simulink model "smm_gait_control"  (R2018b)
settings: configuration reference "Configuration1khz" (kept outside this file)
InitFcn:
  | addpath('./functions/')
  | addpath('./policies/')
  | control_params
values from neighbouring files (symbols this model uses):
  rest = extract_policy_variables('policies/rest.mat')    [control_params.m]
  run_slow = extract_policy_variables('policies/06_run_reduced.mat')    [control_params.m]
  walk_slow = extract_policy_variables('policies/06_walk.mat')    [control_params.m]
undefined symbols (not defined in the file or in its folder): ctrl, Discrete, initial_dx_estimate, initial_dy_estimate, initial_dz_estimate, initial_z_estimate, sample_time, Time
libraries: simulink x42, ctrlSharedLib x7
(part 3 of 5)

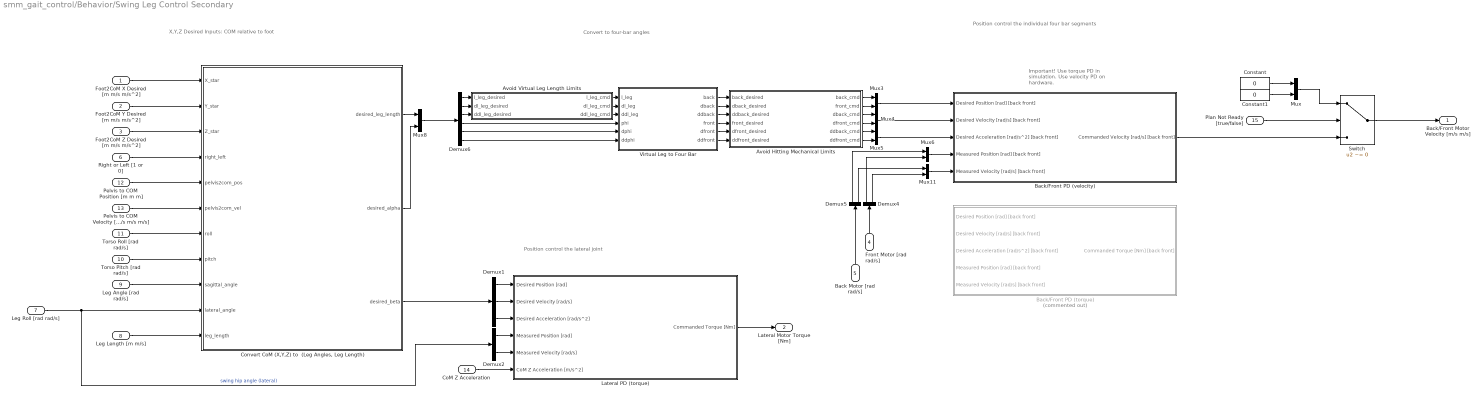
== system smm_gait_control/Behavior/Swing Leg Control Secondary ==
  note: Position control the
      | individual four bar segments
  note: Convert to four-bar angles
  note: X,Y,Z Desired Inputs: COM relative to foot
  note: Important!
      | Use torque PD in simulation.
      | Use velocity PD on hardware.
  note: Position control the lateral joint
  Foot2CoM X Desired [m m/s m/s^2] : Inport
  Foot2CoM Y Desired [m m/s m/s^2] : Inport  Port=2
  Foot2CoM Z Desired [m m/s m/s^2] : Inport  Port=3
  Front Motor [rad rad/s] : Inport  Port=4
  Back Motor [rad rad/s] : Inport  Port=5
  Right or Left [1 or 0] : Inport  Port=6
  Leg Roll [rad rad/s] : Inport  Port=7
  Leg Length [m m/s] : Inport  Port=8
  Leg Angle [rad rad/s] : Inport  Port=9
  Torso Pitch [rad rad/s] : Inport  Port=10
  Torso Roll [rad rad/s] : Inport  Port=11
  Pelvis to COM Position [m m m] : Inport  Port=12
  Pelvis to COM Velocity [m/s m/s m/s] : Inport  Port=13
  CoM Z Acceleration : Inport  Port=14
  Plan Not Ready [true/false] : Inport  Port=15
  Avoid Hitting Mechanical Limits : MATLAB Function  TreatAsAtomicUnit=on
  Avoid Virtual Leg Length Limits : MATLAB Function  TreatAsAtomicUnit=on
  Back/Front PD (torque) : Subsystem  Commented=on
  Back/Front PD (velocity) : Subsystem
  Constant : Constant  Value=0
  Constant1 : Constant  Value=0
  "Convert CoM (X,Y,Z) to  (Leg Angles, Leg Length)" : MATLAB Function  TreatAsAtomicUnit=on
  Demux1 : Demux  Outputs=3
  Demux2 : Demux  Outputs=2
  Demux4 : Demux  Outputs=2
  Demux5 : Demux  Outputs=2
  Demux6 : Demux  Outputs=6
  Lateral PD (torque) : Subsystem
  Mux{,3..6,8,11} (7 alike) : Mux  Inputs=2
  Switch : Switch  Criteria=u2 ~= 0
  Virtual Leg to Four Bar : MATLAB Function  TreatAsAtomicUnit=on
  Back/Front Motor Velocity [m/s m/s] : Outport
  Lateral Motor Torque [Nm] : Outport  Port=2
  wires:
  Demux4/1 -> Mux6/2
  Mux6/1 -> Back/Front PD (velocity)/4(Measured Position [rad] [back front])
  Mux3/1 -> Back/Front PD (velocity)/1(Desired Position [rad] [back front])
  Demux5/2 -> Mux11/1
  Front Motor [rad rad/s]/1 -> Demux4/1
  Mux4/1 -> Back/Front PD (velocity)/2(Desired Velocity [rad/s] [back front])
  Foot2CoM Z Desired [m m/s m/s^2]/1 -> "Convert CoM (X,Y,Z) to  (Leg Angles, Leg Length)"/3(Z_star)
  Demux5/1 -> Mux6/1
  Back Motor [rad rad/s]/1 -> Demux5/1
  Demux6/4 -> Virtual Leg to Four Bar/4(phi)
  Mux11/1 -> Back/Front PD (velocity)/5(Measured Velocity [rad/s] [back front])
  Demux6/6 -> Virtual Leg to Four Bar/6(ddphi)
  Demux6/5 -> Virtual Leg to Four Bar/5(dphi)
  Demux4/2 -> Mux11/2
  Torso Pitch [rad rad/s]/1 -> "Convert CoM (X,Y,Z) to  (Leg Angles, Leg Length)"/8(pitch)
  Torso Roll [rad rad/s]/1 -> "Convert CoM (X,Y,Z) to  (Leg Angles, Leg Length)"/7(roll)
  Right or Left [1 or 0]/1 -> "Convert CoM (X,Y,Z) to  (Leg Angles, Leg Length)"/4(right_left)
  Leg Roll [rad rad/s]/1 -> Demux2/1, "Convert CoM (X,Y,Z) to  (Leg Angles, Leg Length)"/10(lateral_angle)  "swing hip angle (lateral)"
  Leg Angle [rad rad/s]/1 -> "Convert CoM (X,Y,Z) to  (Leg Angles, Leg Length)"/9(sagittal_angle)
  "Convert CoM (X,Y,Z) to  (Leg Angles, Leg Length)"/2(desired_alpha) -> Mux8/2
  Leg Length [m m/s]/1 -> "Convert CoM (X,Y,Z) to  (Leg Angles, Leg Length)"/11(leg_length)
  "Convert CoM (X,Y,Z) to  (Leg Angles, Leg Length)"/1(desired_leg_length) -> Mux8/1
  Mux8/1 -> Demux6/1
  Foot2CoM Y Desired [m m/s m/s^2]/1 -> "Convert CoM (X,Y,Z) to  (Leg Angles, Leg Length)"/2(Y_star)
  Pelvis to COM Position [m m m]/1 -> "Convert CoM (X,Y,Z) to  (Leg Angles, Leg Length)"/5(pelvis2com_pos)
  Pelvis to COM Velocity [m/s m/s m/s]/1 -> "Convert CoM (X,Y,Z) to  (Leg Angles, Leg Length)"/6(pelvis2com_vel)
  "Convert CoM (X,Y,Z) to  (Leg Angles, Leg Length)"/3(desired_beta) -> Demux1/1
  Foot2CoM X Desired [m m/s m/s^2]/1 -> "Convert CoM (X,Y,Z) to  (Leg Angles, Leg Length)"/1(X_star)
  Mux5/1 -> Back/Front PD (velocity)/3(Desired Acceleration [rad/s^2] [back front])
  Demux1/1 -> Lateral PD (torque)/1(Desired Position [rad])
  Demux1/3 -> Lateral PD (torque)/3(Desired Acceleration [rad/s^2])
  Demux1/2 -> Lateral PD (torque)/2(Desired Velocity [rad/s])
  Lateral PD (torque)/1(Commanded Torque [Nm]) -> Lateral Motor Torque [Nm]/1
  Demux2/2 -> Lateral PD (torque)/5(Measured Velocity [rad/s])
  Demux2/1 -> Lateral PD (torque)/4(Measured Position [rad])
  CoM Z Acceleration/1 -> Lateral PD (torque)/6(CoM Z Acceleration [m/s^2])
  Virtual Leg to Four Bar/1(back) -> Avoid Hitting Mechanical Limits/1(back_desired)
  Virtual Leg to Four Bar/2(dback) -> Avoid Hitting Mechanical Limits/2(dback_desired)
  Virtual Leg to Four Bar/3(ddback) -> Avoid Hitting Mechanical Limits/3(ddback_desired)
  Virtual Leg to Four Bar/4(front) -> Avoid Hitting Mechanical Limits/4(front_desired)
  Virtual Leg to Four Bar/5(dfront) -> Avoid Hitting Mechanical Limits/5(dfront_desired)
  Virtual Leg to Four Bar/6(ddfront) -> Avoid Hitting Mechanical Limits/6(ddfront_desired)
  Avoid Hitting Mechanical Limits/1(back_cmd) -> Mux3/1
  Avoid Hitting Mechanical Limits/6(ddfront_cmd) -> Mux5/2
  Avoid Hitting Mechanical Limits/2(front_cmd) -> Mux3/2
  Avoid Hitting Mechanical Limits/3(dback_cmd) -> Mux4/1
  Avoid Hitting Mechanical Limits/4(dfront_cmd) -> Mux4/2
  Avoid Hitting Mechanical Limits/5(ddback_cmd) -> Mux5/1
  Demux6/1 -> Avoid Virtual Leg Length Limits/1(l_leg_desired)
  Demux6/2 -> Avoid Virtual Leg Length Limits/2(dl_leg_desired)
  Demux6/3 -> Avoid Virtual Leg Length Limits/3(ddl_leg_desired)
  Avoid Virtual Leg Length Limits/1(l_leg_cmd) -> Virtual Leg to Four Bar/1(l_leg)
  Avoid Virtual Leg Length Limits/2(dl_leg_cmd) -> Virtual Leg to Four Bar/2(dl_leg)
  Avoid Virtual Leg Length Limits/3(ddl_leg_cmd) -> Virtual Leg to Four Bar/3(ddl_leg)
  Mux/1 -> Switch/1
  Constant/1 -> Mux/1
  Back/Front PD (velocity)/1(Commanded Velocity [rad/s] [back front]) -> Switch/3
  Plan Not Ready [true/false]/1 -> Switch/2
  Constant1/1 -> Mux/2
  Switch/1 -> Back/Front Motor Velocity [m/s m/s]/1

== system smm_gait_control/Behavior/Tranform Sensor Measurements to CoM Acceleration Measurement ==
  note: Important!
      | Include gravitational acceleration.
      | (Not measured by accelerometers)
  Pitch State [rad rad/s] : Inport
  Roll State [rad rad/s] : Inport  Port=2
  Yaw State [rad rad/s] : Inport  Port=3
  Imu Accelerations : Inport  Port=4
  Enabled [true/false] : Inport  Port=5
  R Hip Roll [rad rad/s] : Inport  Port=6
  L Hip Roll [rad rad/s] : Inport  Port=7
  COM Acceleration Measurement : Scope  NumInputPorts=3
  Compute Body Frame Accelerations : Subsystem
  Compute CoM Translational Acceleration : MATLAB Function  TreatAsAtomicUnit=on
  Demux : Demux  Outputs=3
  Demux3 : Demux  Outputs=3
  Estimate Angular Accelerations2 : Subsystem
  Estimate Angular Accelerations3 : Subsystem
  Fcn : Fcn  Expr=u - ctrl.g
  Mux28 : Mux  Inputs=3
  Mux3 : Mux  Inputs=3
  Mux30 : Mux  Inputs=2
  Selector{,1..2,41..42} (5 alike) : Selector  InputPortWidth=2  IndexOptions=Index vector (dialog)  Indices=[2]  OutputSizes=1
  Terminator{3..5,7} (4 alike) : Terminator
  CoM Acceleration [m/s] x3 : Outport
  wires:
  Demux/1 -> COM Acceleration Measurement/1
  Demux/3 -> COM Acceleration Measurement/3
  [enabled] -> Estimate Angular Accelerations2/2(Enabled)
  Yaw State [rad rad/s]/1 -> Selector2/1
  Mux30/1 -> Estimate Angular Accelerations3/1(Angular Velocities [rad/s] x2)
  Demux/2 -> COM Acceleration Measurement/2
  Pitch State [rad rad/s]/1 -> Selector1/1, Compute CoM Translational Acceleration/4(torso_pitch)
  Roll State [rad rad/s]/1 -> Selector/1, Compute CoM Translational Acceleration/3(torso_roll)
  Estimate Angular Accelerations2/1(Angular Accelerations [rad/s^2] x3) -> Compute CoM Translational Acceleration/1(torso_angular_accelerations)
  Compute Body Frame Accelerations/1(accelerations [m/s^2] x3) -> Compute CoM Translational Acceleration/2(imu_translational_accelerations_body)
  Compute CoM Translational Acceleration/5(left_hip_acceleration_yawed) -> Terminator5/1
  Compute CoM Translational Acceleration/2(torso_com_acceleration_yawed) -> Terminator3/1
  Mux28/1 -> Estimate Angular Accelerations2/1(Angular Velocities [rad/s] x3)
  Imu Accelerations/1 -> Compute Body Frame Accelerations/1(imu accelerations x3)
  R Hip Roll [rad rad/s]/1 -> Selector41/1, Compute CoM Translational Acceleration/6(right_hip_roll)
  L Hip Roll [rad rad/s]/1 -> Selector42/1, Compute CoM Translational Acceleration/7(left_hip_roll)
  Selector/1 -> Mux28/1
  Selector1/1 -> Mux28/2
  Selector2/1 -> Mux28/3
  Compute CoM Translational Acceleration/4(right_hip_acceleration_yawed) -> Terminator4/1
  Compute CoM Translational Acceleration/3(pelvis_acceleration_yawed) -> Terminator7/1
  Demux3/1 -> Mux3/1
  Demux3/3 -> Fcn/1
  Fcn/1 -> Mux3/3
  Demux3/2 -> Mux3/2
  Compute CoM Translational Acceleration/1(com_acceleration_yawed) -> Demux3/1
  Selector41/1 -> Mux30/1
  Selector42/1 -> Mux30/2
  Estimate Angular Accelerations3/1(Angular Accelerations [rad/s^2] x2) -> Compute CoM Translational Acceleration/5(hip_roll_accelerations)
  Enabled [true/false]/1 -> [enabled]
  [enabled] -> Estimate Angular Accelerations3/2(Enabled)
  Mux3/1 -> Demux/1, CoM Acceleration [m/s] x3/1

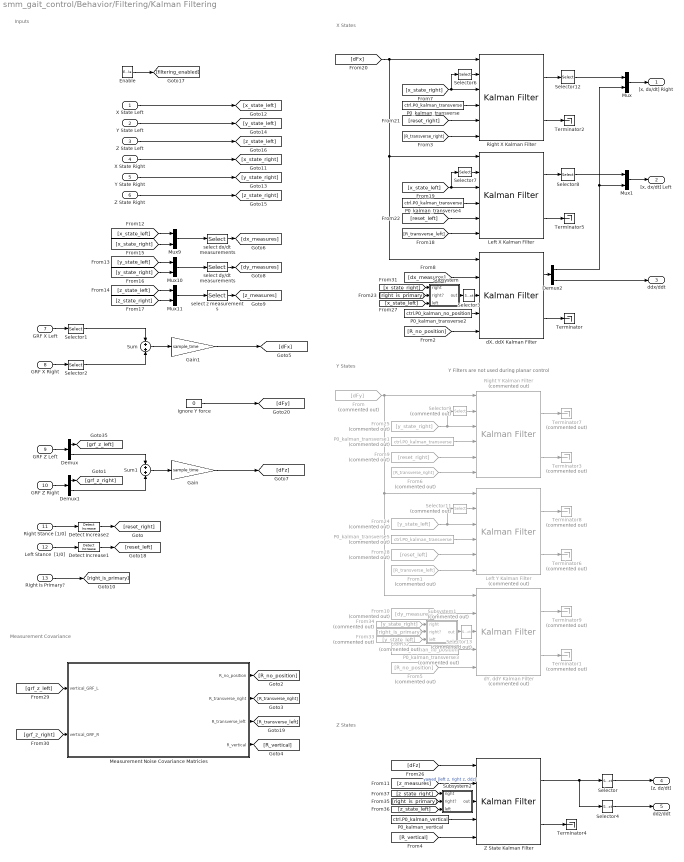
== system smm_gait_control/Behavior/Filtering/Kalman Filtering ==
  note: Y Filters are not used during planar control
  note: Inputs
  note: X States
  note: Y States
  note: Z States
  note: Measurement Covariance
  X State Left : Inport  SampleTime=sample_time
  Y State Left : Inport  Port=2  SampleTime=sample_time
  Z State Left : Inport  Port=3  SampleTime=sample_time
  X State Right : Inport  Port=4  SampleTime=sample_time
  Y State Right : Inport  Port=5  SampleTime=sample_time
  Z State Right : Inport  Port=6  SampleTime=sample_time
  GRF X Left : Inport  Port=7  SampleTime=sample_time
  GRF X Right : Inport  Port=8  SampleTime=sample_time
  GRF Z Left : Inport  Port=9  SampleTime=sample_time
  GRF Z Right : Inport  Port=10  SampleTime=sample_time
  Right Stance [1/0] : Inport  Port=11  PortDimensions=1  SampleTime=sample_time
  Left Stance  [1/0] : Inport  Port=12  PortDimensions=1  SampleTime=sample_time
  Right Is Primary? : Inport  Port=13  SampleTime=sample_time
  Enable : EnablePort  StatesWhenEnabling=reset  ShowOutputPort=on
  Demux : Demux  Outputs=2
  Demux1 : Demux  Outputs=2
  Demux2 : Demux  Outputs=2
  Detect Increase1 : simulink/Logic and Bit Operations/Detect Increase  vinit=0.0  OutDataTypeStr=boolean
  Detect Increase2 : simulink/Logic and Bit Operations/Detect Increase  vinit=0.0  OutDataTypeStr=boolean
  From : From  Commented=on  GotoTag=dFy
  From1 : From  Commented=on  GotoTag=R_transverse_left
  From10 : From  Commented=on  GotoTag=dy_measures
  From24 : From  Commented=on  GotoTag=y_state_left
  From25 : From  Commented=on  GotoTag=y_state_right
  From28 : From  Commented=on  GotoTag=reset_left
  From32 : From  Commented=on  GotoTag=right_is_primary
  From33 : From  Commented=on  GotoTag=y_state_left
  From34 : From  Commented=on  GotoTag=y_state_right
  From5 : From  Commented=on  GotoTag=R_no_position
  From6 : From  Commented=on  GotoTag=R_transverse_right
  From9 : From  Commented=on  GotoTag=reset_right
  Gain : Gain  Gain=sample_time
  Gain1 : Gain  Gain=sample_time
  Ignore Y force : Constant  Value=0
  Left X Kalman Filter : ctrlSharedLib/Kalman Filter  TimeDomain=Discrete-Time  UseCurrentEstimator=on  ModelSource=Individual A, B, C, D matrices  ModelSourceVariable=A_kf  A=ctrl.A_kalman_3rd_order  B=ctrl.B_kalman_3rd_order  C=ctrl.C_kalman_transverse  D=0  NumberOfStates=2  NumberOfInputs=1  NumberOfOutputs=2  InitialEstimateSource=Input port  X0=initial_dx_estimate  P0=P0_kalman_transverse  UseK=off  UseGH=on  NumberOfProcessNoiseInputs=1  G=ctrl.G_kalman_transverse  TimeInvariantG=on  H=0  TimeInvariantH=on  Q=ctrl.Q_kalman_GRFx_difference*sample_time  TimeInvariantQ=on  R=1  TimeInvariantR=off  N=0  TimeInvariantN=on  AddInputPort=on  AddEnablePort=off  ExternalReset=Rising  OutputEstimatedY=off  OutputP=on  Ts=sample_time
      settings: SourceProductBaseCode=CT
  Left Y Kalman Filter : ctrlSharedLib/Kalman Filter  Commented=on  TimeDomain=Discrete-Time  UseCurrentEstimator=on  ModelSource=Individual A, B, C, D matrices  ModelSourceVariable=A_kf  A=ctrl.A_kalman_3rd_order  B=ctrl.B_kalman_3rd_order  C=ctrl.C_kalman_transverse  D=0  NumberOfStates=2  NumberOfInputs=1  NumberOfOutputs=2  InitialEstimateSource=Input port  X0=initial_dy_estimate  P0=P0_kalman_transverse  UseK=off  UseGH=on  NumberOfProcessNoiseInputs=1  G=ctrl.G_kalman_transverse  TimeInvariantG=on  H=0  TimeInvariantH=on  Q=ctrl.Q_kalman_GRFy_difference*sample_time  TimeInvariantQ=on  R=1  TimeInvariantR=off  N=0  TimeInvariantN=on  AddInputPort=on  AddEnablePort=off  ExternalReset=Rising  OutputEstimatedY=off  OutputP=on  Ts=sample_time
      settings: SourceProductBaseCode=CT
  Measurement Noise Covariance Matricies : MATLAB Function  TreatAsAtomicUnit=on
  Mux{,1,9..11} (5 alike) : Mux  Inputs=2
  P0_kalman_transverse : Constant  Value=ctrl.P0_kalman_transverse
  P0_kalman_transverse1 : Constant  Commented=on  Value=ctrl.P0_kalman_transverse
  P0_kalman_transverse2 : Constant  Value=ctrl.P0_kalman_no_position
  P0_kalman_transverse3 : Constant  Commented=on  Value=ctrl.P0_kalman_no_position
  P0_kalman_transverse4 : Constant  Value=ctrl.P0_kalman_transverse
  P0_kalman_transverse5 : Constant  Commented=on  Value=ctrl.P0_kalman_transverse
  P0_kalman_vertical : Constant  Value=ctrl.P0_kalman_vertical
  Right X Kalman Filter : ctrlSharedLib/Kalman Filter  TimeDomain=Discrete-Time  UseCurrentEstimator=on  ModelSource=Individual A, B, C, D matrices  ModelSourceVariable=A_kf  A=ctrl.A_kalman_3rd_order  B=ctrl.B_kalman_3rd_order  C=ctrl.C_kalman_transverse  D=0  NumberOfStates=2  NumberOfInputs=1  NumberOfOutputs=2  InitialEstimateSource=Input port  X0=initial_dx_estimate  P0=P0_kalman_transverse  UseK=off  UseGH=on  NumberOfProcessNoiseInputs=1  G=ctrl.G_kalman_transverse  TimeInvariantG=on  H=0  TimeInvariantH=on  Q=ctrl.Q_kalman_GRFx_difference*sample_time  TimeInvariantQ=on  R=1  TimeInvariantR=off  N=0  TimeInvariantN=on  AddInputPort=on  AddEnablePort=off  ExternalReset=Rising  OutputEstimatedY=off  OutputP=on  Ts=sample_time
      settings: SourceProductBaseCode=CT
  Right Y Kalman Filter : ctrlSharedLib/Kalman Filter  Commented=on  TimeDomain=Discrete-Time  UseCurrentEstimator=on  ModelSource=Individual A, B, C, D matrices  ModelSourceVariable=A_kf  A=ctrl.A_kalman_3rd_order  B=ctrl.B_kalman_3rd_order  C=ctrl.C_kalman_transverse  D=0  NumberOfStates=2  NumberOfInputs=1  NumberOfOutputs=2  InitialEstimateSource=Input port  X0=initial_dy_estimate  P0=P0_kalman_transverse  UseK=off  UseGH=on  NumberOfProcessNoiseInputs=1  G=ctrl.G_kalman_transverse  TimeInvariantG=on  H=0  TimeInvariantH=on  Q=ctrl.Q_kalman_GRFy_difference*sample_time  TimeInvariantQ=on  R=1  TimeInvariantR=off  N=0  TimeInvariantN=on  AddInputPort=on  AddEnablePort=off  ExternalReset=Rising  OutputEstimatedY=off  OutputP=on  Ts=sample_time
      settings: SourceProductBaseCode=CT
  Selector : Selector  InputPortWidth=3  IndexOptions=Index vector (dialog)  Indices=[1 2]  OutputSizes=1
  Selector1 : Selector  InputPortWidth=2  IndexOptions=Index vector (dialog)  Indices=[2]  OutputSizes=1
  Selector11 : Selector  Commented=on  InputPortWidth=3  IndexOptions=Index vector (dialog)  Indices=[1 3]  OutputSizes=1
  Selector12 : Selector  InputPortWidth=3  IndexOptions=Index vector (dialog)  Indices=[1]  OutputSizes=1
  Selector13 : Selector  Commented=on  InputPortWidth=3  IndexOptions=Index vector (dialog)  Indices=[2 3]  OutputSizes=1
  Selector2 : Selector  InputPortWidth=2  IndexOptions=Index vector (dialog)  Indices=[2]  OutputSizes=1
  Selector3 : Selector  InputPortWidth=3  IndexOptions=Index vector (dialog)  Indices=[2 3]  OutputSizes=1
  Selector4 : Selector  InputPortWidth=3  IndexOptions=Index vector (dialog)  Indices=[3]  OutputSizes=1
  Selector6 : Selector  InputPortWidth=3  IndexOptions=Index vector (dialog)  Indices=[1 3]  OutputSizes=1
  Selector7 : Selector  InputPortWidth=3  IndexOptions=Index vector (dialog)  Indices=[1 3]  OutputSizes=1
  Selector8 : Selector  InputPortWidth=3  IndexOptions=Index vector (dialog)  Indices=[1]  OutputSizes=1
  Selector9 : Selector  Commented=on  InputPortWidth=3  IndexOptions=Index vector (dialog)  Indices=[1 3]  OutputSizes=1
  Subsystem : Subsystem
  Subsystem1 : Subsystem  Commented=on
  Subsystem2 : Subsystem
  Sum : Sum  Inputs=+|+
  Sum1 : Sum  Inputs=+|+
  Terminator{,2,4..5} (4 alike) : Terminator
  Terminator{1,3,6..9} (6 alike) : Terminator  Commented=on
  Z State Kalman Filter : ctrlSharedLib/Kalman Filter  TimeDomain=Discrete-Time  UseCurrentEstimator=on  ModelSource=Individual A, B, C, D matrices  ModelSourceVariable=A_kf  A=ctrl.A_kalman_3rd_order  B=ctrl.B_kalman_3rd_order  C=ctrl.C_kalman_vertical  D=0  NumberOfStates=2  NumberOfInputs=1  NumberOfOutputs=2  InitialEstimateSource=Input port  X0=[initial_z_estimate; initial_dz_estimate]  P0=P0_kalman_vertical  UseK=off  UseGH=on  NumberOfProcessNoiseInputs=1  G=ctrl.G_kalman_vertical  TimeInvariantG=on  H=0  TimeInvariantH=on  Q=ctrl.Q_kalman_GRFz_difference*sample_time  TimeInvariantQ=on  R=1  TimeInvariantR=off  N=0  TimeInvariantN=on  AddInputPort=on  AddEnablePort=off  OutputEstimatedY=off  OutputP=on  Ts=sample_time
      settings: SourceProductBaseCode=CT
  "dX, ddX Kalman Filter" : ctrlSharedLib/Kalman Filter  TimeDomain=Discrete-Time  UseCurrentEstimator=on  ModelSource=Individual A, B, C, D matrices  ModelSourceVariable=A_kf  A=ctrl.A_kalman_2nd_order  B=ctrl.B_kalman_2nd_order  C=ctrl.C_kalman_no_position  D=0  NumberOfStates=2  NumberOfInputs=1  NumberOfOutputs=2  InitialEstimateSource=Input port  X0=initial_dx_estimate  P0=P0_kalman_transverse  UseK=off  UseGH=on  NumberOfProcessNoiseInputs=1  G=ctrl.G_kalman_no_position  TimeInvariantG=on  H=0  TimeInvariantH=on  Q=ctrl.Q_kalman_GRFx_difference*sample_time  TimeInvariantQ=on  R=1  TimeInvariantR=off  N=0  TimeInvariantN=on  AddInputPort=on  AddEnablePort=off  OutputEstimatedY=off  OutputP=on  Ts=sample_time
      settings: SourceProductBaseCode=CT
  "dY, ddY Kalman Filter" : ctrlSharedLib/Kalman Filter  Commented=on  TimeDomain=Discrete-Time  UseCurrentEstimator=on  ModelSource=Individual A, B, C, D matrices  ModelSourceVariable=A_kf  A=ctrl.A_kalman_2nd_order  B=ctrl.B_kalman_2nd_order  C=ctrl.C_kalman_no_position  D=0  NumberOfStates=2  NumberOfInputs=1  NumberOfOutputs=2  InitialEstimateSource=Input port  X0=initial_dx_estimate  P0=P0_kalman_transverse  UseK=off  UseGH=on  NumberOfProcessNoiseInputs=1  G=ctrl.G_kalman_no_position  TimeInvariantG=on  H=0  TimeInvariantH=on  Q=ctrl.Q_kalman_GRFx_difference*sample_time  TimeInvariantQ=on  R=1  TimeInvariantR=off  N=0  TimeInvariantN=on  AddInputPort=on  AddEnablePort=off  OutputEstimatedY=off  OutputP=on  Ts=sample_time
      settings: SourceProductBaseCode=CT
  select dx/dt measurements : Selector  InputPortWidth=6  IndexOptions=Index vector (dialog)  Indices=[2 5 6]  OutputSizes=1
  select dy/dt measurements : Selector  InputPortWidth=6  IndexOptions=Index vector (dialog)  Indices=[2 5 6]  OutputSizes=1
  select z measurements : Selector  InputPortWidth=6  IndexOptions=Index vector (dialog)  Indices=[1 4 6]  OutputSizes=1
  "[x, dx/dt] Right" : Outport
  "[x, dx/dt] Left" : Outport  Port=2
  ddx/ddt : Outport  Port=3
  "[z, dz/dt]" : Outport  Port=4
  ddz/ddt : Outport  Port=5
  wires:
  [R_no_position] -> "dX, ddX Kalman Filter"/5
  P0_kalman_transverse2/1 -> "dX, ddX Kalman Filter"/4
  Subsystem/1(out) -> Selector3/1
  [dx_measures] -> "dX, ddX Kalman Filter"/2
  Z State Kalman Filter/1 -> Selector4/1, Selector/1
  [z_measures] -> Z State Kalman Filter/2  "yawed [left z, right z, ddz]"
  [R_vertical] -> Z State Kalman Filter/5
  [grf_z_right] -> Measurement Noise Covariance Matricies/2(vertical_GRF_R)
  [grf_z_left] -> Measurement Noise Covariance Matricies/1(vertical_GRF_L)
  P0_kalman_transverse1/1 -> Right Y Kalman Filter/4
  [dFz] -> Z State Kalman Filter/1
  P0_kalman_transverse/1 -> Right X Kalman Filter/4
  [dFx] -> Right X Kalman Filter/1, Left X Kalman Filter/1, "dX, ddX Kalman Filter"/1
  Right X Kalman Filter/1 -> Selector12/1
  "dX, ddX Kalman Filter"/2 -> Terminator/1
  [R_transverse_right] -> Right X Kalman Filter/6
  P0_kalman_vertical/1 -> Z State Kalman Filter/4
  "dY, ddY Kalman Filter"/2 -> Terminator1/1
  Subsystem1/1(out) -> Selector13/1
  P0_kalman_transverse3/1 -> "dY, ddY Kalman Filter"/4
  From10/1 -> "dY, ddY Kalman Filter"/2
  Measurement Noise Covariance Matricies/1(R_no_position) -> [R_no_position]
  Measurement Noise Covariance Matricies/2(R_transverse_right) -> [R_transverse_right]
  Measurement Noise Covariance Matricies/4(R_vertical) -> [R_vertical]
  From5/1 -> "dY, ddY Kalman Filter"/5
  From6/1 -> Right Y Kalman Filter/6
  Right Is Primary?/1 -> [right_is_primary]
  Y State Right/1 -> [y_state_right]
  [x_state_left] -> Mux9/1
  [x_state_right] -> Mux9/2
  [y_state_left] -> Mux10/1
  [y_state_right] -> Mux10/2
  [z_state_left] -> Mux11/1
  [z_state_right] -> Mux11/2
  Mux9/1 -> select dx/dt measurements/1
  Mux10/1 -> select dy/dt measurements/1
  Mux11/1 -> select z measurements/1
  select dx/dt measurements/1 -> [dx_measures]
  select dy/dt measurements/1 -> [dy_measures]
  select z measurements/1 -> [z_measures]
  Right X Kalman Filter/2 -> Terminator2/1
  Right Y Kalman Filter/2 -> Terminator3/1
  Z State Kalman Filter/2 -> Terminator4/1
  Enable/1 -> [filtering_enabled]
  [x_state_right] -> Selector6/1, Right X Kalman Filter/3
  Selector6/1 -> Right X Kalman Filter/2
  Selector7/1 -> Left X Kalman Filter/2
  [x_state_left] -> Left X Kalman Filter/3, Selector7/1
  [R_transverse_left] -> Left X Kalman Filter/6
  P0_kalman_transverse4/1 -> Left X Kalman Filter/4
  Left X Kalman Filter/1 -> Selector8/1
  Left X Kalman Filter/2 -> Terminator5/1
  [reset_right] -> Right X Kalman Filter/5
  [reset_left] -> Left X Kalman Filter/5
  From9/1 -> Right Y Kalman Filter/5
  From25/1 -> Selector9/1, Right Y Kalman Filter/3
  Selector9/1 -> Right Y Kalman Filter/2
  Selector11/1 -> Left Y Kalman Filter/2
  From24/1 -> Left Y Kalman Filter/3, Selector11/1
  From28/1 -> Left Y Kalman Filter/5
  Left Y Kalman Filter/2 -> Terminator6/1
  From1/1 -> Left Y Kalman Filter/6
  From/1 -> Right Y Kalman Filter/1, Left Y Kalman Filter/1, "dY, ddY Kalman Filter"/1
  P0_kalman_transverse5/1 -> Left Y Kalman Filter/4
  Right Stance [1/0]/1 -> Detect Increase2/1
  Left Stance  [1/0]/1 -> Detect Increase1/1
  Detect Increase1/1 -> [reset_left]
  Detect Increase2/1 -> [reset_right]
  GRF X Left/1 -> Selector1/1
  GRF X Right/1 -> Selector2/1
  Sum/1 -> Gain1/1
  Measurement Noise Covariance Matricies/3(R_transverse_left) -> [R_transverse_left]
  GRF Z Left/1 -> Demux/1
  GRF Z Right/1 -> Demux1/1
  Sum1/1 -> Gain/1
  Demux/1 -> [grf_z_left]
  Demux1/1 -> [grf_z_right]
  Selector1/1 -> Sum/1
  Selector2/1 -> Sum/2
  Demux/2 -> Sum1/1
  Demux1/2 -> Sum1/2
  Gain/1 -> [dFz]
  Gain1/1 -> [dFx]
  Ignore Y force/1 -> [dFy]
  Mux/1 -> "[x, dx/dt] Right"/1
  Selector12/1 -> Mux/1
  Mux1/1 -> "[x, dx/dt] Left"/1
  Selector8/1 -> Mux1/1
  Right Y Kalman Filter/1 -> Terminator7/1
  Left Y Kalman Filter/1 -> Terminator8/1
  "dY, ddY Kalman Filter"/1 -> Terminator9/1
  [x_state_right] -> Subsystem/1(right)
  [right_is_primary] -> Subsystem/2(right?)
  [x_state_left] -> Subsystem/3(left)
  From32/1 -> Subsystem1/2(right?)
  From34/1 -> Subsystem1/1(right)
  From33/1 -> Subsystem1/3(left)
  Selector13/1 -> "dY, ddY Kalman Filter"/3
  Selector3/1 -> "dX, ddX Kalman Filter"/3
  [right_is_primary] -> Subsystem2/2(right?)
  [z_state_right] -> Subsystem2/1(right)
  [z_state_left] -> Subsystem2/3(left)
  Subsystem2/1(out) -> Z State Kalman Filter/3
  Selector/1 -> "[z, dz/dt]"/1
  Demux2/1 -> Mux1/2, Mux/2
  Demux2/2 -> ddx/ddt/1
  Selector4/1 -> ddz/ddt/1
  "dX, ddX Kalman Filter"/1 -> Demux2/1
  Z State Left/1 -> [z_state_left]
  Y State Left/1 -> [y_state_left]
  X State Left/1 -> [x_state_left]
  Z State Right/1 -> [z_state_right]
  X State Right/1 -> [x_state_right]

== system smm_gait_control/Behavior/Filtering/Subsystem2 ==
  right : Inport
  right? : Inport  Port=2
  left : Inport  Port=3
  Switch : Switch  Criteria=u2 ~= 0
  out : Outport
  wires:
  right/1 -> Switch/1
  right?/1 -> Switch/2
  left/1 -> Switch/3
  Switch/1 -> out/1

== system smm_gait_control/Behavior/Motion Planner/Hold Value ==
  In : Inport
  Enable : EnablePort
  Out : Outport  InitialOutput=0
  wires:
  In/1 -> Out/1

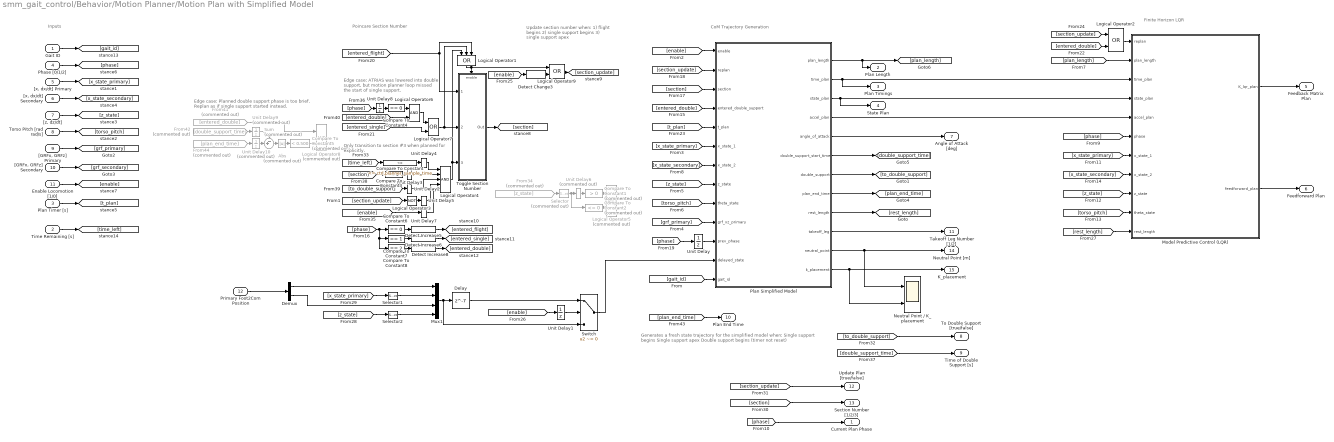
== system smm_gait_control/Behavior/Motion Planner/Motion Plan with Simplified Model ==
  note: Edge case: ATRIAS was lowered into
      | double support, but motion planner loop
      | missed the start of single support.
  note: Update section number when:
      | 1) flight begins
      | 2) single support begins
      | 3) single support apex
  note: Inputs
  note: Poincare Section Number
  note: CoM Trajectory Generation
  note: Finite Horizon LQR
  note: Generates a fresh state trajectory for the simplified model when:
      | Single support begins
      | Single support apex
      | Double support begins (timer not reset)
  note: Only transition to section #3 when planned
      | for explicitly.
  note: Edge case: Planned double support phase is too brief.
      | Replan as if single support started instead.
  Gait ID : Inport
  Time Remaining [s] : Inport  Port=2
  Plan Timer [s] : Inport  Port=3
  Phase [0/1/2] : Inport  Port=4
  "[x, dx/dt] Primary" : Inport  Port=5
  "[x, dx/dt] Secondary" : Inport  Port=6
  "[z, dz/dt]" : Inport  Port=7
  Torso Pitch [rad rad/s] : Inport  Port=8
  "[GRFx, GRFz] Primary" : Inport  Port=9
  "[GRFx, GRFz] Secondary" : Inport  Port=10
  Enable Locomotion [1/0] : Inport  Port=11
  Primary Foot2Com Position : Inport  Port=12
  Abs : Abs  Commented=on
  Compare To Constant : simulink/Logic and Bit Operations/Compare To Constant  relop=<=  const=ctrl.planner_sample_time  OutDataTypeStr=boolean
  Compare To Constant1 : simulink/Logic and Bit Operations/Compare To Constant  Commented=on  relop=>  const=0  OutDataTypeStr=boolean
  Compare To Constant2 : simulink/Logic and Bit Operations/Compare To Constant  Commented=on  relop=<=  const=0  OutDataTypeStr=boolean
  Compare To Constant3 : simulink/Logic and Bit Operations/Compare To Constant  relop===  const=2  OutDataTypeStr=boolean
  Compare To Constant4 : simulink/Logic and Bit Operations/Compare To Constant  relop===  const=0  OutDataTypeStr=boolean
  Compare To Constant5 : simulink/Logic and Bit Operations/Compare To Constant  Commented=on  relop=<  const=0.500  OutDataTypeStr=boolean
  Compare To Constant6 : simulink/Logic and Bit Operations/Compare To Constant  relop===  const=0  OutDataTypeStr=boolean
  Compare To Constant7 : simulink/Logic and Bit Operations/Compare To Constant  relop===  const=1  OutDataTypeStr=boolean
  Compare To Constant8 : simulink/Logic and Bit Operations/Compare To Constant  relop===  const=2  OutDataTypeStr=boolean
  Delay : Delay  DelayLength=7
  Demux : Demux  Outputs=2
  Detect Change3 : simulink/Logic and Bit Operations/Detect Change  vinit=0  OutDataTypeStr=boolean
  Detect Increase5 : simulink/Logic and Bit Operations/Detect Increase  vinit=1  OutDataTypeStr=boolean
  Detect Increase6 : simulink/Logic and Bit Operations/Detect Increase  vinit=0.0  OutDataTypeStr=boolean
  Detect Increase8 : simulink/Logic and Bit Operations/Detect Increase  vinit=0.0  OutDataTypeStr=boolean
  From34 : From  Commented=on  GotoTag=z_state
  From41 : From  Commented=on  GotoTag=entered_double
  From42 : From  Commented=on  GotoTag=double_support_time
  From44 : From  Commented=on  GotoTag=plan_end_time
  Logical Operator1 : Logic  Operator=OR  Inputs=3  AllPortsSameDT=off  OutDataTypeStr=boolean
  Logical Operator2 : Logic  Operator=OR  AllPortsSameDT=off  OutDataTypeStr=boolean
  Logical Operator3 : Logic  Operator=NOT  Inputs=4  AllPortsSameDT=off  OutDataTypeStr=boolean
  Logical Operator4 : Logic  Inputs=5  AllPortsSameDT=off  OutDataTypeStr=boolean
  Logical Operator5 : Logic  Commented=on  AllPortsSameDT=off  OutDataTypeStr=boolean
  Logical Operator6 : Logic  AllPortsSameDT=off  OutDataTypeStr=boolean
  Logical Operator7 : Logic  Operator=OR  AllPortsSameDT=off  OutDataTypeStr=boolean
  Logical Operator8 : Logic  Commented=on  AllPortsSameDT=off  OutDataTypeStr=boolean
  Logical Operator9 : Logic  Operator=OR  AllPortsSameDT=off  OutDataTypeStr=boolean
  Model Predictive Control (LQR) : MATLAB Function  TreatAsAtomicUnit=on
  Mux1 : Mux
  Neutral Point / K_placement : Scope  NumInputPorts=2
  Plan Simplified Model : MATLAB Function  TreatAsAtomicUnit=on
  Selector : Selector  Commented=on  InputPortWidth=2  IndexOptions=Index vector (dialog)  Indices=[2]  OutputSizes=1
  Selector1 : Selector  InputPortWidth=2  IndexOptions=Index vector (dialog)  Indices=[2]  OutputSizes=1
  Selector2 : Selector  InputPortWidth=2  IndexOptions=Index vector (dialog)  Indices=[2]  OutputSizes=1
  Sum : Sum  Commented=on  Inputs=-+|
  Switch : Switch  Criteria=u2 ~= 0
  Toggle Section Number : Subsystem  TreatAsAtomicUnit=on
  Unit Delay{,1..5,7..8} (8 alike) : UnitDelay  SampleTime=-1
  Unit Delay10 : UnitDelay  Commented=on  SampleTime=-1
  Unit Delay6 : UnitDelay  Commented=on  SampleTime=-1
  Unit Delay9 : UnitDelay  Commented=on  SampleTime=-1
  Current Plan Phase : Outport
  Plan Length : Outport  Port=2
  Plan Timings : Outport  Port=3
  State Plan : Outport  Port=4
  Feedback Matrix Plan : Outport  Port=5
  Feedforward Plan : Outport  Port=6
  Angle of Attack [deg] : Outport  Port=7
  To Double Support [true/false] : Outport  Port=8
  Time of Double Support [s] : Outport  Port=9
  Plan End Time : Outport  Port=10
  Takeoff Leg Number [1/2] : Outport  Port=11
  Update Plan [true/false] : Outport  Port=12
  Section Number [1/2/3] : Outport  Port=13
  Neutral Point [m] : Outport  Port=14
  K_placement : Outport  Port=15
  wires:
  "[GRFx, GRFz] Secondary"/1 -> [grf_secondary]
  "[GRFx, GRFz] Primary"/1 -> [grf_primary]
  Plan Timer [s]/1 -> [t_plan]
  "[x, dx/dt] Secondary"/1 -> [x_state_secondary]
  Torso Pitch [rad rad/s]/1 -> [torso_pitch]
  "[x, dx/dt] Primary"/1 -> [x_state_primary]
  "[z, dz/dt]"/1 -> [z_state]
  [enable] -> Plan Simplified Model/1(enable)
  [x_state_primary] -> Plan Simplified Model/6(x_state_1)
  [x_state_secondary] -> Plan Simplified Model/7(x_state_2)
  [z_state] -> Plan Simplified Model/8(z_state)
  [torso_pitch] -> Plan Simplified Model/9(theta_state)
  [grf_primary] -> Plan Simplified Model/10(grf_xz_primary)
  Logical Operator7/1 -> Logical Operator1/2, Toggle Section Number/2(2)
  [entered_flight] -> Toggle Section Number/1(1), Logical Operator1/3
  Logical Operator1/1 -> Logical Operator9/1, Toggle Section Number/Enable
  [phase] -> Model Predictive Control (LQR)/6(phase)
  [x_state_primary] -> Model Predictive Control (LQR)/7(x_state_1)
  [x_state_secondary] -> Model Predictive Control (LQR)/8(x_state_2)
  [z_state] -> Model Predictive Control (LQR)/9(z_state)
  [torso_pitch] -> Model Predictive Control (LQR)/10(theta_state)
  Plan Simplified Model/4(accel_plan) -> Model Predictive Control (LQR)/5(accel_plan)
  Plan Simplified Model/3(state_plan) -> Model Predictive Control (LQR)/4(state_plan), State Plan/1
  Plan Simplified Model/2(time_plan) -> Model Predictive Control (LQR)/3(time_plan), Plan Timings/1
  Model Predictive Control (LQR)/1(K_lqr_plan) -> Feedback Matrix Plan/1
  Model Predictive Control (LQR)/2(feedforward_plan) -> Feedforward Plan/1
  Plan Simplified Model/5(angle_of_attack) -> Angle of Attack [deg]/1
  [entered_double] -> Logical Operator2/2
  Toggle Section Number/1(Out) -> [section]
  [section] -> Plan Simplified Model/3(section)
  Compare To Constant6/1 -> Detect Increase5/1
  [phase] -> Compare To Constant8/1, Compare To Constant7/1, Compare To Constant6/1
  Compare To Constant7/1 -> Detect Increase6/1
  Compare To Constant8/1 -> Detect Increase8/1
  Detect Increase5/1 -> [entered_flight]
  Detect Increase6/1 -> [entered_single]
  Detect Increase8/1 -> [entered_double]
  [entered_double] -> Plan Simplified Model/4(entered_double_support)
  [t_plan] -> Plan Simplified Model/5(t_plan)
  Plan Simplified Model/7(double_support) -> [to_double_support]
  Plan Simplified Model/6(double_support_start_time) -> [double_support_time]
  Gait ID/1 -> [gait_id]
  [gait_id] -> Plan Simplified Model/13(gait_id)
  Plan Simplified Model/8(plan_end_time) -> [plan_end_time]
  [phase] -> Unit Delay/1
  Unit Delay/1 -> Plan Simplified Model/11(prev_phase)
  Primary Foot2Com Position/1 -> Demux/1
  [x_state_primary] -> Selector1/1
  [z_state] -> Selector2/1
  Selector2/1 -> Mux1/4
  Selector1/1 -> Mux1/2
  Demux/1 -> Mux1/1
  Demux/2 -> Mux1/3
  Switch/1 -> Plan Simplified Model/12(delayed_state)
  [enable] -> Unit Delay1/1
  Unit Delay1/1 -> Switch/2
  Delay/1 -> Switch/1
  Mux1/1 -> Switch/3, Delay/1
  Plan Simplified Model/10(takeoff_leg) -> Takeoff Leg Number [1/2]/1
  Plan Simplified Model/9(rest_length) -> [rest_length]
  [rest_length] -> Model Predictive Control (LQR)/11(rest_length)
  [section] -> Section Number [1/2/3]/1
  [to_double_support] -> To Double Support [true/false]/1
  [double_support_time] -> Time of Double Support [s]/1
  [section] -> Compare To Constant3/1
  [time_left] -> Compare To Constant/1
  Logical Operator4/1 -> Logical Operator1/1, Toggle Section Number/3(3)
  Plan Simplified Model/11(neutral_point) -> Neutral Point / K_placement/1, Neutral Point [m]/1
  Plan Simplified Model/12(k_placement) -> Neutral Point / K_placement/2, K_placement/1
  [section_update] -> Plan Simplified Model/2(replan)
  [section_update] -> Update Plan [true/false]/1
  Logical Operator2/1 -> Model Predictive Control (LQR)/1(replan)
  Enable Locomotion [1/0]/1 -> [enable]
  Phase [0/1/2]/1 -> [phase]
  Detect Change3/1 -> Logical Operator9/2
  [enable] -> Detect Change3/1
  Logical Operator9/1 -> [section_update]
  [section_update] -> Logical Operator2/1
  Plan Simplified Model/1(plan_length) -> [plan_length], Plan Length/1
  [plan_length] -> Model Predictive Control (LQR)/2(plan_length)
  [phase] -> Current Plan Phase/1
  Time Remaining [s]/1 -> [time_left]
  [to_double_support] -> Unit Delay2/1
  Compare To Constant3/1 -> Unit Delay3/1
  Compare To Constant/1 -> Unit Delay4/1
  Unit Delay4/1 -> Logical Operator4/1
  Unit Delay3/1 -> Logical Operator4/2
  Unit Delay2/1 -> Logical Operator4/3
  [section_update] -> Logical Operator3/1
  Logical Operator3/1 -> Unit Delay5/1
  Unit Delay5/1 -> Logical Operator4/4
  From34/1 -> Selector/1
  Unit Delay6/1 -> Compare To Constant1/1
  Selector/1 -> Compare To Constant2/1, Unit Delay6/1
  Compare To Constant1/1 -> Logical Operator5/1
  Compare To Constant2/1 -> Logical Operator5/2
  [enable] -> Unit Delay7/1
  Unit Delay7/1 -> Logical Operator4/5
  [phase] -> Unit Delay8/1
  Unit Delay8/1 -> Compare To Constant4/1
  Compare To Constant4/1 -> Logical Operator6/1
  [entered_double] -> Logical Operator6/2
  [entered_single] -> Logical Operator7/2
  Logical Operator6/1 -> Logical Operator7/1
  From42/1 -> Unit Delay9/1
  [plan_end_time] -> Plan End Time/1
  Unit Delay9/1 -> Sum/1
  Unit Delay10/1 -> Sum/2
  Sum/1 -> Abs/1
  Abs/1 -> Compare To Constant5/1
  Compare To Constant5/1 -> Logical Operator8/2
  From41/1 -> Logical Operator8/1
  From44/1 -> Unit Delay10/1

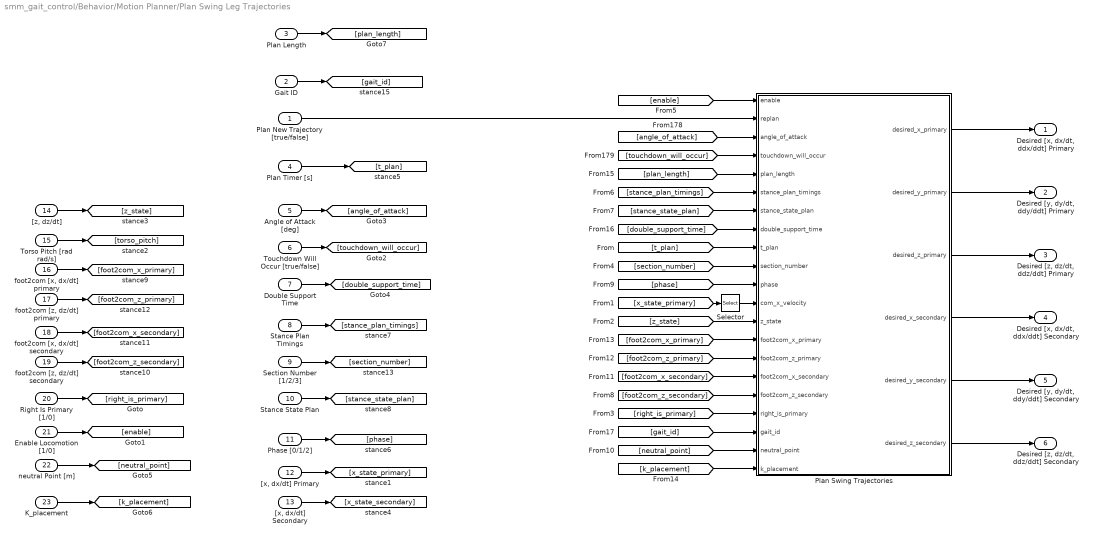
== system smm_gait_control/Behavior/Motion Planner/Plan Swing Leg Trajectories ==
  Plan New Trajectory [true/false] : Inport
  Gait ID : Inport  Port=2
  Plan Length : Inport  Port=3
  Plan Timer [s] : Inport  Port=4
  Angle of Attack [deg] : Inport  Port=5
  Touchdown Will Occur [true/false] : Inport  Port=6
  "Double Support Time " : Inport  Port=7
  Stance Plan Timings : Inport  Port=8
  Section Number [1/2/3] : Inport  Port=9
  Stance State Plan : Inport  Port=10
  Phase [0/1/2] : Inport  Port=11
  "[x, dx/dt] Primary" : Inport  Port=12
  "[x, dx/dt] Secondary" : Inport  Port=13
  "[z, dz/dt]" : Inport  Port=14
  Torso Pitch [rad rad/s] : Inport  Port=15
  "foot2com [x, dx/dt] primary" : Inport  Port=16
  "foot2com [z, dz/dt] primary" : Inport  Port=17
  "foot2com [x, dx/dt] secondary" : Inport  Port=18
  "foot2com [z, dz/dt] secondary" : Inport  Port=19
  Right Is Primary [1/0] : Inport  Port=20
  Enable Locomotion [1/0] : Inport  Port=21
  neutral Point [m] : Inport  Port=22
  K_placement : Inport  Port=23
  Plan Swing Trajectories : MATLAB Function  TreatAsAtomicUnit=on
  Selector : Selector  InputPortWidth=2  IndexOptions=Index vector (dialog)  Indices=[2]  OutputSizes=1
  "Desired [x, dx/dt, ddx/ddt] Primary" : Outport
  "Desired [y, dy/dt, ddy/ddt] Primary" : Outport  Port=2
  "Desired [z, dz/dt, ddz/ddt] Primary" : Outport  Port=3
  "Desired [x, dx/dt, ddx/ddt] Secondary" : Outport  Port=4
  "Desired [y, dy/dt, ddy/ddt] Secondary" : Outport  Port=5
  "Desired [z, dz/dt, ddz/ddt] Secondary" : Outport  Port=6
  wires:
  Plan Timer [s]/1 -> [t_plan]
  Phase [0/1/2]/1 -> [phase]
  "[x, dx/dt] Secondary"/1 -> [x_state_secondary]
  Plan New Trajectory [true/false]/1 -> Plan Swing Trajectories/2(replan)
  Torso Pitch [rad rad/s]/1 -> [torso_pitch]
  "[x, dx/dt] Primary"/1 -> [x_state_primary]
  "[z, dz/dt]"/1 -> [z_state]
  Plan Swing Trajectories/1(desired_x_primary) -> "Desired [x, dx/dt, ddx/ddt] Primary"/1
  Plan Swing Trajectories/2(desired_y_primary) -> "Desired [y, dy/dt, ddy/ddt] Primary"/1
  Plan Swing Trajectories/3(desired_z_primary) -> "Desired [z, dz/dt, ddz/ddt] Primary"/1
  Plan Swing Trajectories/4(desired_x_secondary) -> "Desired [x, dx/dt, ddx/ddt] Secondary"/1
  Plan Swing Trajectories/5(desired_y_secondary) -> "Desired [y, dy/dt, ddy/ddt] Secondary"/1
  Plan Swing Trajectories/6(desired_z_secondary) -> "Desired [z, dz/dt, ddz/ddt] Secondary"/1
  Right Is Primary [1/0]/1 -> [right_is_primary]
  Enable Locomotion [1/0]/1 -> [enable]
  "foot2com [x, dx/dt] secondary"/1 -> [foot2com_x_secondary]
  "foot2com [x, dx/dt] primary"/1 -> [foot2com_x_primary]
  "foot2com [z, dz/dt] secondary"/1 -> [foot2com_z_secondary]
  "foot2com [z, dz/dt] primary"/1 -> [foot2com_z_primary]
  [enable] -> Plan Swing Trajectories/1(enable)
  [t_plan] -> Plan Swing Trajectories/9(t_plan)
  [phase] -> Plan Swing Trajectories/11(phase)
  [z_state] -> Plan Swing Trajectories/13(z_state)
  [foot2com_x_primary] -> Plan Swing Trajectories/14(foot2com_x_primary)
  [foot2com_z_primary] -> Plan Swing Trajectories/15(foot2com_z_primary)
  [foot2com_x_secondary] -> Plan Swing Trajectories/16(foot2com_x_secondary)
  [foot2com_z_secondary] -> Plan Swing Trajectories/17(foot2com_z_secondary)
  [right_is_primary] -> Plan Swing Trajectories/18(right_is_primary)
  [angle_of_attack] -> Plan Swing Trajectories/3(angle_of_attack)
  [touchdown_will_occur] -> Plan Swing Trajectories/4(touchdown_will_occur)
  Touchdown Will Occur [true/false]/1 -> [touchdown_will_occur]
  Angle of Attack [deg]/1 -> [angle_of_attack]
  Stance Plan Timings/1 -> [stance_plan_timings]
  Stance State Plan/1 -> [stance_state_plan]
  [stance_state_plan] -> Plan Swing Trajectories/7(stance_state_plan)
  [stance_plan_timings] -> Plan Swing Trajectories/6(stance_plan_timings)
  "Double Support Time "/1 -> [double_support_time]
  [double_support_time] -> Plan Swing Trajectories/8(double_support_time)
  Gait ID/1 -> [gait_id]
  [gait_id] -> Plan Swing Trajectories/19(gait_id)
  [x_state_primary] -> Selector/1
  Selector/1 -> Plan Swing Trajectories/12(com_x_velocity)
  Section Number [1/2/3]/1 -> [section_number]
  [section_number] -> Plan Swing Trajectories/10(section_number)
  neutral Point [m]/1 -> [neutral_point]
  K_placement/1 -> [k_placement]
  [neutral_point] -> Plan Swing Trajectories/20(neutral_point)
  [k_placement] -> Plan Swing Trajectories/21(k_placement)
  Plan Length/1 -> [plan_length]
  [plan_length] -> Plan Swing Trajectories/5(plan_length)

== system smm_gait_control/Behavior/Swing Leg Control Primary/Back//Front PD (torque) ==
  Desired Position [rad] [back front] : Inport
  Desired Velocity [rad/s] [back front] : Inport  Port=2
  Desired Acceleration [rad/s^2] [back front] : Inport  Port=3
  Measured Position [rad] [back front] : Inport  Port=4
  Measured Velocity [rad/s] [back front] : Inport  Port=5
  Back / Front Position Tracking : Scope  NumInputPorts=2
  Back / Front Velocity Tracking : Scope  NumInputPorts=2
  Feedback / Feedforward : Scope  NumInputPorts=2
  Kp_SEA_Trajectory : Constant  Value=ctrl.kp_torque_swing
  Kp_SEA_Trajectory1 : Constant  Value=ctrl.kd_torque_swing
  Kp_SEA_Trajectory2 : Constant  Value=ctrl.i_motor
  Mux{1..2,12..13} (4 alike) : Mux  Inputs=2
  Product1 : Product
  Product2 : Product
  Product3 : Product
  Selector{,1..3} (4 alike) : Selector  InputPortWidth=2  IndexOptions=Index vector (dialog)  Indices=[1]  OutputSizes=1
  Selector{4..5,7..8} (4 alike) : Selector  InputPortWidth=2  IndexOptions=Index vector (dialog)  Indices=[2]  OutputSizes=1
  Sum1 : Sum  Inputs=|+-
  Sum2 : Sum  Inputs=|++
  Sum7 : Sum  Inputs=|+-
  Sum9 : Sum  Inputs=++|
  Commanded Torque [Nm] [back front] : Outport
  wires:
  Product3/1 -> Sum2/2, Feedback / Feedforward/2
  Kp_SEA_Trajectory2/1 -> Product3/1
  Desired Acceleration [rad/s^2] [back front]/1 -> Product3/2
  Sum2/1 -> Commanded Torque [Nm] [back front]/1
  Sum9/1 -> Sum2/1, Feedback / Feedforward/1
  Kp_SEA_Trajectory1/1 -> Product2/2
  Sum1/1 -> Product2/1
  Kp_SEA_Trajectory/1 -> Product1/2
  Measured Position [rad] [back front]/1 -> Selector4/1, Selector/1, Sum7/2
  Sum7/1 -> Product1/1
  Product1/1 -> Sum9/1
  Mux13/1 -> Back / Front Position Tracking/1
  Desired Position [rad] [back front]/1 -> Selector5/1, Selector1/1, Sum7/1
  Mux2/1 -> Back / Front Position Tracking/2
  Selector/1 -> Mux13/1
  Selector1/1 -> Mux13/2
  Selector5/1 -> Mux2/2
  Selector4/1 -> Mux2/1
  Desired Velocity [rad/s] [back front]/1 -> Selector8/1, Selector3/1, Sum1/1
  Product2/1 -> Sum9/2
  Measured Velocity [rad/s] [back front]/1 -> Sum1/2, Selector2/1, Selector7/1
  Mux1/1 -> Back / Front Velocity Tracking/1
  Selector2/1 -> Mux1/1
  Selector7/1 -> Mux12/1
  Mux12/1 -> Back / Front Velocity Tracking/2
  Selector8/1 -> Mux12/2
  Selector3/1 -> Mux1/2

== system smm_gait_control/Behavior/Swing Leg Control Primary/Back//Front PD (velocity) ==
  Desired Position [rad] [back front] : Inport
  Desired Velocity [rad/s] [back front] : Inport  Port=2
  Desired Acceleration [rad/s^2] [back front] : Inport  Port=3
  Measured Position [rad] [back front] : Inport  Port=4
  Measured Velocity [rad/s] [back front] : Inport  Port=5
  Back / Front PositionTracking : Scope  NumInputPorts=2
  Back / Front Velocity Tracking : Scope  NumInputPorts=2
  Feedback / Feedforward : Scope  NumInputPorts=2
  Feedforward Gain : Gain
  Kp_SEA_Trajectory : Constant  Value=ctrl.kp_velocity_swing
  Mux{1..2,12..13} (4 alike) : Mux  Inputs=2
  Product1 : Product
  Selector{,1..3} (4 alike) : Selector  InputPortWidth=2  IndexOptions=Index vector (dialog)  Indices=[1]  OutputSizes=1
  Selector{4..5,7..8} (4 alike) : Selector  InputPortWidth=2  IndexOptions=Index vector (dialog)  Indices=[2]  OutputSizes=1
  Sum7 : Sum  Inputs=|+-
  Sum9 : Sum
  Terminator : Terminator
  Commanded Velocity [rad/s] [back front] : Outport
  wires:
  Selector3/1 -> Mux1/2
  Selector8/1 -> Mux12/2
  Mux12/1 -> Back / Front Velocity Tracking/2
  Selector7/1 -> Mux12/1
  Selector2/1 -> Mux1/1
  Mux1/1 -> Back / Front Velocity Tracking/1
  Measured Velocity [rad/s] [back front]/1 -> Selector2/1, Selector7/1
  Desired Acceleration [rad/s^2] [back front]/1 -> Terminator/1
  Feedforward Gain/1 -> Sum9/2, Feedback / Feedforward/2
  Desired Velocity [rad/s] [back front]/1 -> Selector3/1, Selector8/1, Feedforward Gain/1
  Selector4/1 -> Mux2/1
  Selector5/1 -> Mux2/2
  Selector1/1 -> Mux13/2
  Selector/1 -> Mux13/1
  Mux2/1 -> Back / Front PositionTracking/2
  Desired Position [rad] [back front]/1 -> Sum7/1, Selector1/1, Selector5/1
  Mux13/1 -> Back / Front PositionTracking/1
  Product1/1 -> Sum9/1, Feedback / Feedforward/1
  Sum7/1 -> Product1/1
  Measured Position [rad] [back front]/1 -> Sum7/2, Selector/1, Selector4/1
  Sum9/1 -> Commanded Velocity [rad/s] [back front]/1
  Kp_SEA_Trajectory/1 -> Product1/2

== system smm_gait_control/Behavior/Swing Leg Control Primary/Lateral PD (torque) ==
  note: (Approximation)
      | This is the lateral torque generated due to the relative
      | acceleration of the motor around the pelvis. Only
      | approximate vertical components are used in the
      | calculation. The lateral components are small.
  Desired Position [rad] : Inport
  Desired Velocity [rad/s] : Inport  Port=2
  Desired Acceleration [rad/s^2] : Inport  Port=3
  Measured Position [rad] : Inport  Port=4
  Measured Velocity [rad/s] : Inport  Port=5
  CoM Z Acceleration [m/s^2] : Inport  Port=6
  Feedback / Feedforward : Scope  NumInputPorts=2
  Kp_SEA_Trajectory : Constant  Value=ctrl.kp_lateral_swing
  Kp_SEA_Trajectory1 : Constant  Value=ctrl.kd_lateral_swing
  Kp_SEA_Trajectory2 : Constant  Value=ctrl.i_lateral_about_pelvis
  Kp_SEA_Trajectory3 : Constant  Value=ctrl.lateral_offset
  Kp_SEA_Trajectory4 : Constant  Value=(ctrl.m_leg_motor + ctrl.m_leg)
  Kp_SEA_Trajectory5 : Constant  Value=-ctrl.g
  Mux13 : Mux  Inputs=2
  Mux2 : Mux  Inputs=2
  Position / Velocity Tracking : Scope  NumInputPorts=2
  Product1 : Product
  Product2 : Product
  Product3 : Product
  Product4 : Product  Inputs=3
  Sum1 : Sum  Inputs=|+-
  Sum2 : Sum  Inputs=|++
  Sum3 : Sum  Inputs=|++
  Sum4 : Sum  Inputs=|+-
  Sum7 : Sum  Inputs=|+-
  Sum9 : Sum  Inputs=++|
  Commanded Torque [Nm] : Outport
  wires:
  Sum4/1 -> Product4/1
  CoM Z Acceleration [m/s^2]/1 -> Sum4/2
  Kp_SEA_Trajectory5/1 -> Sum4/1
  Kp_SEA_Trajectory3/1 -> Product4/2
  Kp_SEA_Trajectory4/1 -> Product4/3
  Product4/1 -> Sum3/2
  Product3/1 -> Sum3/1
  Measured Velocity [rad/s]/1 -> Sum1/2, Mux2/1
  Product2/1 -> Sum9/2
  Desired Velocity [rad/s]/1 -> Sum1/1, Mux2/2
  Mux2/1 -> Position / Velocity Tracking/2
  Desired Position [rad]/1 -> Sum7/1, Mux13/2
  Mux13/1 -> Position / Velocity Tracking/1
  Product1/1 -> Sum9/1
  Sum7/1 -> Product1/1
  Measured Position [rad]/1 -> Sum7/2, Mux13/1
  Kp_SEA_Trajectory/1 -> Product1/2
  Sum1/1 -> Product2/1
  Kp_SEA_Trajectory1/1 -> Product2/2
  Sum9/1 -> Feedback / Feedforward/1, Sum2/1
  Sum2/1 -> Commanded Torque [Nm]/1
  Desired Acceleration [rad/s^2]/1 -> Product3/2
  Kp_SEA_Trajectory2/1 -> Product3/1
  Sum3/1 -> Feedback / Feedforward/2, Sum2/2

== system smm_gait_control/Behavior/Swing Leg Control Secondary/Back//Front PD (torque) ==
  Desired Position [rad] [back front] : Inport
  Desired Velocity [rad/s] [back front] : Inport  Port=2
  Desired Acceleration [rad/s^2] [back front] : Inport  Port=3
  Measured Position [rad] [back front] : Inport  Port=4
  Measured Velocity [rad/s] [back front] : Inport  Port=5
  Back / Front Position Tracking : Scope  NumInputPorts=2
  Back / Front Velocity Tracking : Scope  NumInputPorts=2
  Feedback / Feedforward : Scope  NumInputPorts=2
  Kp_SEA_Trajectory : Constant  Value=ctrl.kp_torque_swing
  Kp_SEA_Trajectory1 : Constant  Value=ctrl.kd_torque_swing
  Kp_SEA_Trajectory2 : Constant  Value=ctrl.i_motor
  Mux{1..2,12..13} (4 alike) : Mux  Inputs=2
  Product1 : Product
  Product2 : Product
  Product3 : Product
  Selector{,1..3} (4 alike) : Selector  InputPortWidth=2  IndexOptions=Index vector (dialog)  Indices=[1]  OutputSizes=1
  Selector{4..5,7..8} (4 alike) : Selector  InputPortWidth=2  IndexOptions=Index vector (dialog)  Indices=[2]  OutputSizes=1
  Sum1 : Sum  Inputs=|+-
  Sum2 : Sum  Inputs=|++
  Sum7 : Sum  Inputs=|+-
  Sum9 : Sum  Inputs=++|
  Commanded Torque [Nm] [back front] : Outport
  wires:
  Selector3/1 -> Mux1/2
  Selector8/1 -> Mux12/2
  Mux12/1 -> Back / Front Velocity Tracking/2
  Selector7/1 -> Mux12/1
  Selector2/1 -> Mux1/1
  Mux1/1 -> Back / Front Velocity Tracking/1
  Measured Velocity [rad/s] [back front]/1 -> Selector7/1, Selector2/1, Sum1/2
  Product2/1 -> Sum9/2
  Desired Velocity [rad/s] [back front]/1 -> Sum1/1, Selector3/1, Selector8/1
  Selector4/1 -> Mux2/1
  Selector5/1 -> Mux2/2
  Selector1/1 -> Mux13/2
  Selector/1 -> Mux13/1
  Mux2/1 -> Back / Front Position Tracking/2
  Desired Position [rad] [back front]/1 -> Sum7/1, Selector1/1, Selector5/1
  Mux13/1 -> Back / Front Position Tracking/1
  Product1/1 -> Sum9/1
  Sum7/1 -> Product1/1
  Measured Position [rad] [back front]/1 -> Sum7/2, Selector/1, Selector4/1
  Kp_SEA_Trajectory/1 -> Product1/2
  Sum1/1 -> Product2/1
  Kp_SEA_Trajectory1/1 -> Product2/2
  Sum9/1 -> Feedback / Feedforward/1, Sum2/1
  Sum2/1 -> Commanded Torque [Nm] [back front]/1
  Desired Acceleration [rad/s^2] [back front]/1 -> Product3/2
  Kp_SEA_Trajectory2/1 -> Product3/1
  Product3/1 -> Sum2/2, Feedback / Feedforward/2
